simulink library "ClosedFormIK_Lib"  (R2024b)
settings: Solver=VariableStepAuto  StartTime=0.0  StopTime=10.0  RelTol=1e-3
settings Model: Creator=pepev  LastModifiedBy=pepev

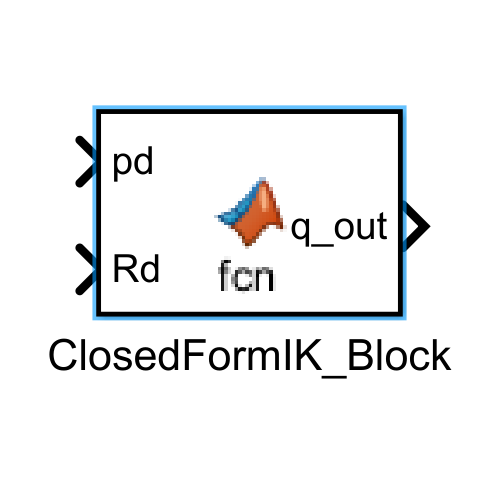
[thumbnail: Simulink's stored preview of the top-level diagram]
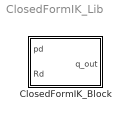
== system ClosedFormIK_Lib ==
  ClosedFormIK_Block : MATLAB Function  TreatAsAtomicUnit=on

== matlab function ClosedFormIK_Lib/ClosedFormIK_Block ==
  data: pd input; q_out output; Rd input
function q_out = fcn(pd, Rd)
    %#codegen
    coder.extrinsic('ClosedFormIK');

    % Preallocate output
    q_out = zeros(6,1);

    % Call your closed-form IK function
    q_out = ClosedFormIK(pd, Rd);

end
